simulink model "easyDU"  (Simulink 7.5)
settings: Solver=ode45  StartTime=-1  StopTime=10.0  RelTol=1e-3
settings Model: Creator=Dranik_win  LastModifiedBy=Dranik_win

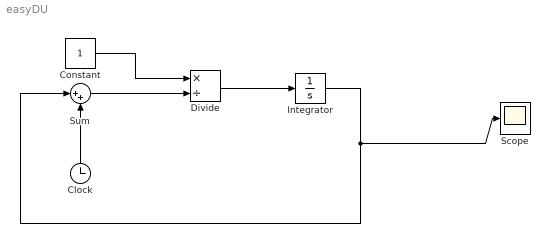
== system easyDU ==
  Clock : Clock
      settings: Decimation=10
  Constant : Constant  OutDataType=fixdt(1, 16)  OutScaling=2^0
  Divide : Product  Inputs=*/  OutDataType=fixdt(1, 16)  OutScaling=2^-10
  Integrator : Integrator
  Scope : Scope
  Sum : Sum  Inputs=|++  OutDataType=fixdt(1, 16)  OutScaling=2^0
  wires:
  Clock/1 -> Sum/2
  Sum/1 -> Divide/2
  Constant/1 -> Divide/1
  Divide/1 -> Integrator/1
  Integrator/1 -> Sum/1, Scope/1
